simulink model "ev_range"  (R2025a)
settings: Solver=VariableStepAuto  StartTime=0.0  StopTime=2500  RelTol=1e-3
values from neighbouring files (symbols this model uses):
  m = 1500    [drivetrain.m]    (also in project_parameters.m = 1400)
libraries: autolibshared x1
settings Model: Creator=DELL  LastModifiedBy=DELL

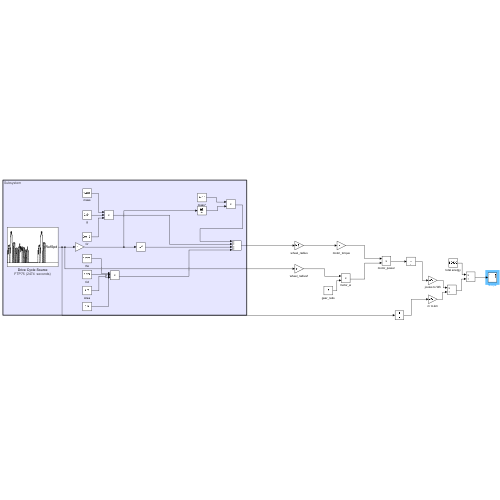
[thumbnail: Simulink's stored preview of the top-level diagram]
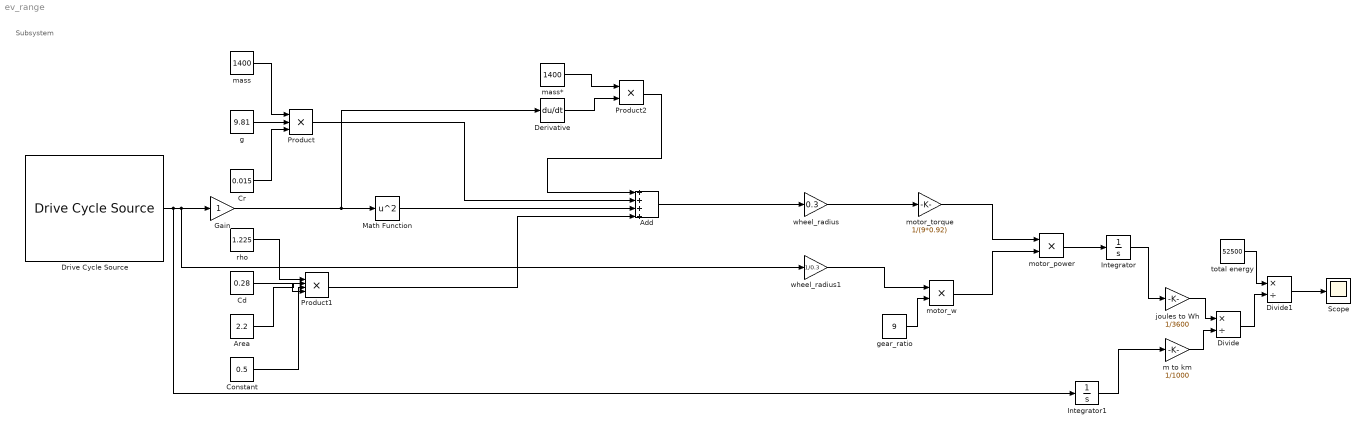
== system ev_range ==
  note: Subsystem
  Add : Sum  Inputs=++++
  Area : Constant  Value=2.2
  Cd : Constant  Value=0.28
  Constant : Constant  Value=0.5
  Cr : Constant  Value=0.015
  Derivative : Derivative
  Divide : Product  Inputs=*/
  Divide1 : Product  Inputs=*/
  Drive Cycle Source : autolibshared/Drive Cycle Source  cycleVar=FTP75  fileVar=cycleFTP75.mat  tfinal="2474  seconds"  cycleRepeat=off  outAccPort=off  outGearPort=off  gearList=No gear data  t_wot1=5  xdot_woto=0  xdot_wot1=30  t_wot2=20  xdot_wot2=0  t_wotend=30  srcUnit=m/s  outUnit=m/s  srcAccUnit=m/s/s  outAccUnit=m/s^2  dt=0  aMode=1  faultOption=off  velBnd=2  velBndUnit=mph  inUnit=m/s  timeBnd=1  failOption=off  stopSim=off  maxFaultCnt=10  maxFaultTime=2  maxTotFaultTime=15  traceOption=off  dtTrace=1  traceWindow=10  lastDCname=FTP75  lastOutUnit=mph  lastDT=0  lastTB=1  lastSB=2  forceCalcBound=off
  Gain : Gain
  Integrator : Integrator
  Integrator1 : Integrator
  Math Function : Math  Operator=square
  Product : Product  Inputs=3
  Product1 : Product  Inputs=4
  Product2 : Product
  Scope : Scope
      settings: ActiveDisplayYMinimum=51.462773655284423  ActiveDisplayYMaximum=612.68053436315392
  g : Constant  Value=9.81
  gear_ratio : Constant  Value=9
  joules to Wh : Gain  Gain=1/3600
  m to km : Gain  Gain=1/1000
  mass : Constant  Value=1400
  mass* : Constant  Value=1400
  motor_power : Product
  motor_torque : Gain  Gain=1/(9*0.92)
  motor_w : Product
  rho : Constant  Value=1.225
  total energy : Constant  Value=52500
  wheel_radius : Gain  Gain=0.3
  wheel_radius1 : Gain  Gain=1/0.3
  wires:
  Constant/1 -> Product1/3
  mass*/1 -> Product2/1
  Drive Cycle Source/1 -> Integrator1/1, wheel_radius1/1, Gain/1
  gear_ratio/1 -> motor_w/2
  rho/1 -> Product1/1
  Math Function/1 -> Add/3
  wheel_radius1/1 -> motor_w/1
  mass/1 -> Product/1
  motor_w/1 -> motor_power/2
  Area/1 -> Product1/2
  Cr/1 -> Product/3
  Derivative/1 -> Product2/2
  g/1 -> Product/2
  Cd/1 -> Product1/4
  Gain/1 -> Derivative/1, Math Function/1
  Product1/1 -> Add/4
  Add/1 -> wheel_radius/1
  Product/1 -> Add/2
  wheel_radius/1 -> motor_torque/1
  Product2/1 -> Add/1
  motor_torque/1 -> motor_power/1
  motor_power/1 -> Integrator/1
  Integrator/1 -> joules to Wh/1
  Integrator1/1 -> m to km/1
  joules to Wh/1 -> Divide/1
  m to km/1 -> Divide/2
  total energy/1 -> Divide1/1
  Divide/1 -> Divide1/2
  Divide1/1 -> Scope/1
